simulink model "drone_HyEQ"  (R2025b)
settings: Solver=VariableStepAuto  StartTime=0.0  StopTime=T  RelTol=1e-3
values from neighbouring files (symbols this model uses):
  J = 100    [init.m]
  T = 100    [init.m]
  x0 = zeros(14,1)    [init.m]
libraries: HyEQ_Library x2, simulink_extras x1
settings Model: Creator=jenniferkouassi  LastModifiedBy=jenniferkouassi
settings DebuggingCC: AlgebraicLoopMsg=none

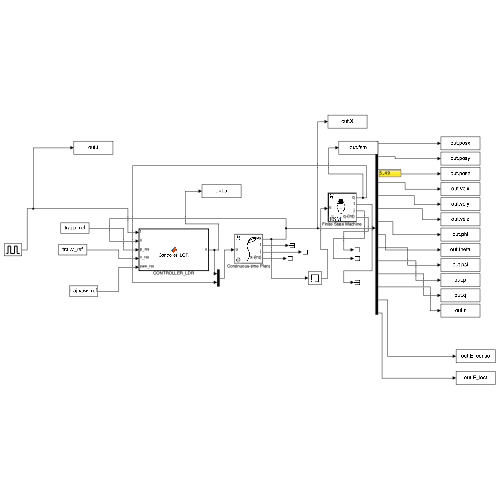
[thumbnail: Simulink's stored preview of the top-level diagram]
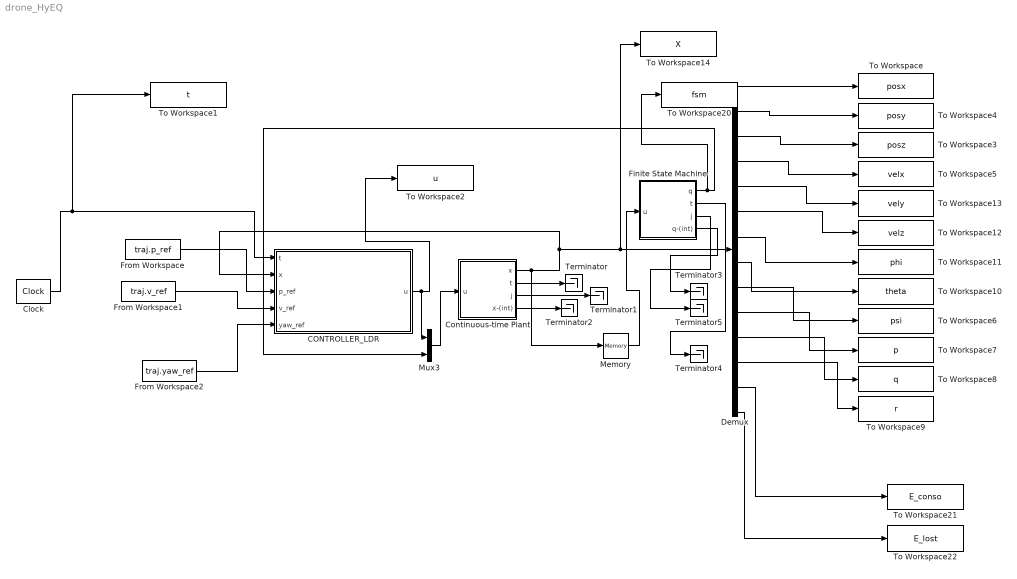
== system drone_HyEQ ==
  CONTROLLER_LDR : MATLAB Function  TreatAsAtomicUnit=on
  Clock : simulink_extras/Flip Flops/Clock  period=120
  Continuous-time Plant : Subsystem  LoadFcn=set_param(gcb,'LinkStatus','none')  mask(Continuous Process){z0=x0, input_dim=[5, 1], parameters=[], T=T}
      mask prompts: z0 "Initial State (column vector)"; input_dim "Input dimension (nonnegative integer)"; T "Flow Horizon (nonnegative real)"
      mask help:
      | To define the continuous process:
      | 1. Select the block,
      | 2. "Look inside" the block: Either open the context menu and select Mask > Look Under Mask, or click the arrow in the bottom-left corner of the block.
      | 3. Edit the "flow map f" block to define the continuous dynamics.
      | 4. Edit the "flow set C" block to define the region where the continuous process is allowed to flow.
      mask init:
      | state_dim = size(z0, 1);
      settings: CopyFcn=|
      | set_param(gcb,'LinkStatus','none'),
      | set_param(gcs, 'MaxStep', 'MaxStep', 'RelTol', 'RelTol','StopTime', 'T')
      mask Help: eval hybrid.internal.openHelp('Example_vehicle_on_path')
      mask TypeOptions T: Integrator System/T
      mask DialogControl Control2 Prompt: CPS Components Documentation
      mask DialogControl Control2 Callback: hybrid.internal.openHelp('CPS_Components')
      mask DialogControl ParameterGroupVar Prompt: Configuration
      mask Display:
      | image('Cplant.jpg')
      | port_label('output', 1, 'x')
      | port_label('output', 2, 't')
      | port_label('output', 3, 'j')
      | port_label('output', 4, 'x-(int)')
      | port_label('input', 1, 'u')
  Demux : Demux  Outputs=14
  Finite State Machine : Subsystem  LoadFcn=set_param(gcb,'LinkStatus','none')  mask(Finite State Machine (FSM)){q0=1, input_dim=14, T=T, J=J}
      mask prompts: q0 "Initial state (column vector)"; input_dim "Input dimension (nonnegative integer)"; T "Flow Horizon (nonnegative real)"; J "Jump Horizon (nonnegative integer)"
      mask help:
      | To define the FSM:
      | 1. Select the block,
      | 2. "Look inside" the block: Either open the context menu and select Mask > Look Under Mask, or click the arrow in the bottom-left corner of the block.
      | 3. Edit the flow set C, jump set D, and jump map g.
      mask init:
      | state_dim = numel(q0);
      settings: CopyFcn=|
      | set_param(gcb,'LinkStatus','none'),
      | set_param(gcs, 'MaxStep', 'MaxStep', 'RelTol', 'RelTol','StopTime', 'T')
      mask Help: eval hybrid.internal.openHelp('CPS_finite_state_machine')
      mask TypeOptions T: Integrator System/T
      mask TypeOptions J: Integrator System/J
      mask DialogControl Control2 Prompt: CPS Components Documentation
      mask DialogControl Control2 Callback: hybrid.internal.openHelp('CPS_Components')
      mask DialogControl Container4 Prompt: Configuration
      mask Display:
      | image('FSM.jpg')
      | port_label('output', 1, 'q')
      | port_label('output', 2, 't')
      | port_label('output', 3, 'j')
      | port_label('output', 4, 'q-(int)')
      | port_label('input', 1, 'u')
  From Workspace : FromWorkspace  VariableName=traj.p_ref  OutputAfterFinalValue=Holding final value
  From Workspace1 : FromWorkspace  VariableName=traj.v_ref  OutputAfterFinalValue=Holding final value
  From Workspace2 : FromWorkspace  VariableName=traj.yaw_ref
  Memory : Memory
  Mux3 : Mux  Inputs=2
  Terminator{,1..5} (6 alike) : Terminator
  To Workspace : ToWorkspace  VariableName=posx  SaveFormat=Timeseries
  To Workspace1 : ToWorkspace  VariableName=t  SaveFormat=Timeseries
  To Workspace10 : ToWorkspace  VariableName=theta  SaveFormat=Timeseries
  To Workspace11 : ToWorkspace  VariableName=phi  SaveFormat=Timeseries
  To Workspace12 : ToWorkspace  VariableName=velz  SaveFormat=Timeseries
  To Workspace13 : ToWorkspace  VariableName=vely  SaveFormat=Timeseries
  To Workspace14 : ToWorkspace  VariableName=X  SaveFormat=Timeseries
  To Workspace2 : ToWorkspace  VariableName=u  SaveFormat=Timeseries
      settings: Save2DSignal=2-D array (concatenate along first dimension)
  To Workspace20 : ToWorkspace  VariableName=fsm  SaveFormat=Timeseries  SampleTime=-1
      settings: Save2DSignal=2-D array (concatenate along first dimension)
  To Workspace21 : ToWorkspace  VariableName=E_conso  SaveFormat=Timeseries  SampleTime=-1
      settings: Save2DSignal=2-D array (concatenate along first dimension)
  To Workspace22 : ToWorkspace  VariableName=E_lost  SaveFormat=Timeseries  SampleTime=-1
      settings: Save2DSignal=2-D array (concatenate along first dimension)
  To Workspace3 : ToWorkspace  VariableName=posz  SaveFormat=Timeseries
  To Workspace4 : ToWorkspace  VariableName=posy  SaveFormat=Timeseries
      settings: Save2DSignal=2-D array (concatenate along first dimension)
  To Workspace5 : ToWorkspace  VariableName=velx  SaveFormat=Timeseries
  To Workspace6 : ToWorkspace  VariableName=psi  SaveFormat=Timeseries
  To Workspace7 : ToWorkspace  VariableName=p  SaveFormat=Timeseries
  To Workspace8 : ToWorkspace  VariableName=q  SaveFormat=Timeseries
  To Workspace9 : ToWorkspace  VariableName=r  SaveFormat=Timeseries
  wires:
  Clock/1 -> To Workspace1/1, CONTROLLER_LDR/1(t)
  Continuous-time Plant/1(x) -> Memory/1, CONTROLLER_LDR/2(x), To Workspace14/1, Demux/1
  From Workspace/1 -> CONTROLLER_LDR/3(p_ref)
  From Workspace1/1 -> CONTROLLER_LDR/4(v_ref)
  From Workspace2/1 -> CONTROLLER_LDR/5(yaw_ref)
  CONTROLLER_LDR/1(u) -> Mux3/1, To Workspace2/1
  Continuous-time Plant/2(t) -> Terminator/1
  Continuous-time Plant/3(j) -> Terminator1/1
  Continuous-time Plant/4(x-(int)) -> Terminator2/1
  Demux/12 -> To Workspace9/1
  Demux/11 -> To Workspace8/1
  Demux/10 -> To Workspace7/1
  Demux/9 -> To Workspace6/1
  Demux/8 -> To Workspace10/1
  Demux/7 -> To Workspace11/1
  Demux/6 -> To Workspace12/1
  Demux/5 -> To Workspace13/1
  Demux/4 -> To Workspace5/1
  Demux/3 -> To Workspace3/1
  Demux/2 -> To Workspace4/1
  Demux/1 -> To Workspace/1
  Finite State Machine/4(q-(int)) -> Terminator3/1
  Finite State Machine/3(j) -> Terminator5/1
  Finite State Machine/2(t) -> Terminator4/1
  Finite State Machine/1(q) -> To Workspace20/1, Mux3/2
  Mux3/1 -> Continuous-time Plant/1(u)
  Memory/1 -> Finite State Machine/1(u)
  Demux/13 -> To Workspace21/1
  Demux/14 -> To Workspace22/1

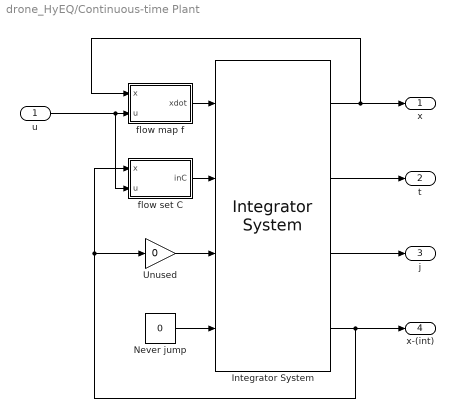
== system drone_HyEQ/Continuous-time Plant ==
  u : Inport  PortDimensions=input_dim
  Integrator System : HyEQ_Library/Other/Integrator System  Priority=2  T=T  J=1  x0=z0  rule=1
      settings: SourceProductName=Hybrid Equations Toolbox
  Never jump : Constant  Value=0
  Unused : Gain  Gain=0
  flow map f : MATLAB Function  TreatAsAtomicUnit=on
  flow set C : MATLAB Function  TreatAsAtomicUnit=on
  x : Outport  PortDimensions=state_dim
  t : Outport  Port=2  PortDimensions=1
  j : Outport  Port=3  PortDimensions=1
  x-(int) : Outport  Port=4  PortDimensions=state_dim
  wires:
  Unused/1 -> Integrator System/3
  Never jump/1 -> Integrator System/4
  u/1 -> flow map f/2(u), flow set C/2(u)
  Integrator System/3 -> j/1
  Integrator System/2 -> t/1
  flow set C/1(inC) -> Integrator System/2
  Integrator System/1 -> x/1, flow map f/1(x)
  Integrator System/4 -> x-(int)/1, flow set C/1(x), Unused/1
  flow map f/1(xdot) -> Integrator System/1

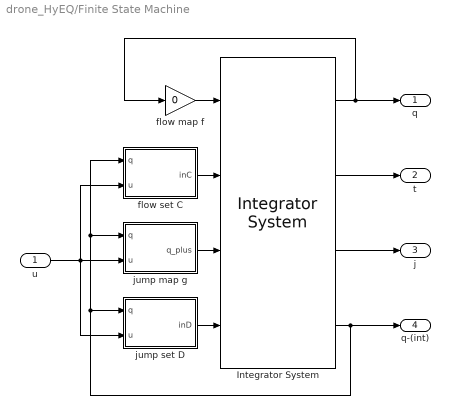
== system drone_HyEQ/Finite State Machine ==
  u : Inport  PortDimensions=input_dim
  Integrator System : HyEQ_Library/Other/Integrator System  Priority=2  T=T  J=J  x0=q0  rule=1
      settings: SourceProductName=Hybrid Equations Toolbox
  flow map f : Gain  Gain=0
  flow set C : MATLAB Function  TreatAsAtomicUnit=on
  jump map g : MATLAB Function  TreatAsAtomicUnit=on
  jump set D : MATLAB Function  TreatAsAtomicUnit=on
  q : Outport  PortDimensions=state_dim
  t : Outport  Port=2  PortDimensions=1
  j : Outport  Port=3  PortDimensions=1
  q-(int) : Outport  Port=4  PortDimensions=state_dim
  wires:
  jump map g/1(q_plus) -> Integrator System/3
  jump set D/1(inD) -> Integrator System/4
  u/1 -> jump map g/2(u), jump set D/2(u), flow set C/2(u)
  Integrator System/3 -> j/1
  Integrator System/2 -> t/1
  flow set C/1(inC) -> Integrator System/2
  Integrator System/1 -> q/1, flow map f/1
  Integrator System/4 -> q-(int)/1, flow set C/1(q), jump map g/1(q), jump set D/1(q)
  flow map f/1 -> Integrator System/1

== matlab function drone_HyEQ/CONTROLLER_LDR ==
  data: t input; u output size=[4, 1]; x input; p_ref input; v_ref input; yaw_ref input; P parameter
function u = Controller_LQR(t, x, p_ref, v_ref, yaw_ref, P)
%CONTROLLER_LQR Cascaded LQR controller for quadcopter
%   x   = [px py pz vx vy vz phi theta psi p q r]'
%   P   = parameter struct (contains precomputed K_pos and K_att)

%% --- Outer loop: Position control (x,y) -> desired accelerations ---
x_pos = x(1:6);
xr_pos = [p_ref; v_ref];

% Calcul de l'accélération désirée pour x et y avec LQR
u_pos = -P.K_pos * (x_pos - xr_pos);

%% --- Contrôle vertical (évite la chute) ---
z    = x(3);      % position actuelle
vz   = x(6);      % vitesse verticale
zref = p_ref(3);  % position désirée
vzref = v_ref(3); % vitesse désirée

Kpz = 6;          % gain proportionnel vertical
Kdz = 3;          % gain dérivé vertical
az_des = Kpz*(zref - z) + Kdz*(vzref - vz);  % accélération verticale désirée

F_total = P.m * (P.g + az_des);              % poussée totale (hover + correction)
F_total = min(max(F_total, 0), 3*P.m*P.g);   % limite pour éviter la saturation

%% --- Map desired acceleration to desired roll/pitch ---
psi = x(9);
phi_des   = (1/P.g) * (u_pos(1)*sin(psi) - u_pos(2)*cos(psi));
theta_des = (1/P.g) * (u_pos(1)*cos(psi) + u_pos(2)*sin(psi));

%% --- Inner loop: Attitude control (phi, theta, psi) -> torques ---
x_att = x(7:12);
xr_att = [phi_des; theta_des; yaw_ref; 0; 0; 0];
tau = -P.K_att * (x_att - xr_att);

% Saturation des couples
tau = max(min(tau, P.tau_max), -P.tau_max);

%% --- Sortie du contrôleur ---
u = [F_total; tau];

end

== matlab function drone_HyEQ/Finite State Machine/flow set C ==
  data: q input size=state_dim; u input size=input_dim; inC output size=1
function inC = C(q, u)

% Force q to be an exact integer but KEEP IT DOUBLE
q = round(q);

alt = u(3);

switch q
    case 1
        inC = (alt <= 1.5);

    case 2
        inC = (alt > 0.5 && alt <= 2.5);

    case 3
        inC = (alt > 1.5 && alt <= 4.0);

    case 4
        inC = (alt > 2.5);

    otherwise
        inC = false;
end

end

== matlab function drone_HyEQ/Finite State Machine/jump map g ==
  data: q input size=state_dim; u input size=input_dim; q_plus output size=state_dim
function q_plus = g(q, u)

% Ensure q is integer-valued but REMAINING double
q = round(q);

alt = u(3);

switch q

    case 1
        q_plus = 2;

    case 2
        if alt > 1.5
            q_plus = 3;
        else
            q_plus = 1;
        end

    case 3
        if alt > 3.0
            q_plus = 4;
        else
            q_plus = 2;
        end

    case 4
        if alt < 2.5
            q_plus = 3;
        else
            q_plus = 4;
        end

    otherwise
        q_plus = 1;

end

end

== matlab function drone_HyEQ/Finite State Machine/jump set D ==
  data: q input size=state_dim; u input size=input_dim; inD output size=1
function inD = D(q, u)

% Keep q DOUBLE but integer-valued
q = round(q);

alt = u(3);

switch q
    case 1
        inD = (alt > 1.0);

    case 2
        inD = (alt > 2.0);

    case 3
        inD = (alt > 3.0);

    case 4
        inD = (alt < 2.0);

    otherwise
        inD = false;
end

end

== matlab function drone_HyEQ/Continuous-time Plant/flow map f ==
  data: x input size=state_dim; xdot output size=state_dim; u input size=input_dim; P parameter
function xdot = f(x, u, P)
% DYNAMIQUE COMPLETE DU DRONE
% AVEC TRAÎNÉE MULTI-SURFACES + COUPLES AÉRODYNAMIQUES + ÉNERGIE

%% === 1. Décomposition des entrées ===
u_cmd = u(1:4);    % [u1 ; tau_x ; tau_y ; tau_z]
mode_FSM = u(5);   % q = 1 → calme, 2 → vent léger, 3 → rafales, 4 → tempête

%% === 2. Vent selon FSM (déterministe, pas de randn) ===
%% === 2. Vent selon FSM (4 niveaux : calme → tempête) ===

pos_x = x(1);
pos_y = x(2);
pos_z = x(3);

% Turbulence pseudo-aléatoire déterministe (pas de randn)
rafale_x =  1.2 * sin(0.6 * pos_x) + 0.8 * cos(1.1 * pos_y);
rafale_y =  0.6 * sin(0.9 * pos_y) + 0.5 * cos(1.3 * pos_z);
rafale_z =  0.3 * sin(0.5 * pos_z) + 0.3 * cos(0.7 * pos_x);

switch mode_FSM      % q = 1 / 2 / 3 / 4

    case 1  % --- Calme ---
        V_air = [0; 0; 0];

    case 2  % --- Vent léger ---
        V_air = [ 3 + 0.4*rafale_x ;
                  0.5*rafale_y ;
                  0.2*rafale_z ];

    case 3  % --- Rafales modérées ---
        V_air = [ 6 + 1.2*rafale_x ;
                      1*rafale_y ;
                  0.6*rafale_z ];

    case 4  % --- Tempête ---
        V_air = [ 10 + 2.0*rafale_x ;
                        2*rafale_y ;
                        1*rafale_z ];

    otherwise
        V_air = [0;0;0];

end

%% === 3. États ===
vx = x(4); vy = x(5); vz = x(6);
phi = x(7); theta = x(8); psi = x(9);
p = x(10); q = x(11); r = x(12);

V_drone = [vx; vy; vz];
V_rel   = V_air - V_drone;     % vitesse du vent relative

%% === 4. Aérodynamique multisurface (forces + moments) ===
F_vent = [0; 0; 0];
M_vent = [0; 0; 0];

%% --- Face avant (X+) ---
Vn = V_rel(1);
F = -0.5 * P.rho * P.Sx_front * P.Cd * Vn * abs(Vn) * [1;0;0];
F_vent = F_vent + F;
M_vent = M_vent + cross(P.r_cp_x, F);

%% --- Face arrière (X−) ---
Vn = -V_rel(1);
F = -0.5 * P.rho * P.Sx_back * P.Cd * Vn * abs(Vn) * [-1;0;0];
F_vent = F_vent + F;
M_vent = M_vent + cross(P.r_cp_mx, F);

%% --- Face droite (Y+) ---
Vn = V_rel(2);
F = -0.5 * P.rho * P.Sy_right * P.Cd * Vn * abs(Vn) * [0;1;0];
F_vent = F_vent + F;
M_vent = M_vent + cross(P.r_cp_y, F);

%% --- Face gauche (Y−) ---
Vn = -V_rel(2);
F = -0.5 * P.rho * P.Sy_left * P.Cd * Vn * abs(Vn) * [0;-1;0];
F_vent = F_vent + F;
M_vent = M_vent + cross(P.r_cp_my, F);

%% --- Face dessus (Z+) ---
Vn = V_rel(3);
F = -0.5 * P.rho * P.Sz_top * P.Cd * Vn * abs(Vn) * [0;0;1];
F_vent = F_vent + F;
M_vent = M_vent + cross(P.r_cp_z, F);

%% --- Face dessous (Z−) ---
Vn = -V_rel(3);
F = -0.5 * P.rho * P.Sz_bottom * P.Cd * Vn * abs(Vn) * [0;0;-1];
F_vent = F_vent + F;
M_vent = M_vent + cross(P.r_cp_mz, F);

%% === 5. Rotation (matrice R du corps vers monde) ===
cphi = cos(phi);  sphi = sin(phi);
cth  = cos(theta); sth  = sin(theta);
cpsi = cos(psi);  spsi = sin(psi);

R = [ cth*cpsi,  sphi*sth*cpsi - cphi*spsi,  cphi*sth*cpsi + sphi*spsi;
      cth*spsi,  sphi*sth*spsi + cphi*cpsi,  cphi*sth*spsi - sphi*cpsi;
     -sth,       sphi*cth,                  cphi*cth ];

%% === 6. Translation ===
u1 = u_cmd(1);

p_dot = [vx; vy; vz];

v_dot = (1/P.m) * (R*[0;0;u1] + F_vent) - [0;0;P.g];

%% === 7. Angles ===
E = [1,  sphi*tan(theta),  cphi*tan(theta);
     0,  cphi,            -sphi;
     0,  sphi/cth,         cphi/cth];

eul_dot = E * [p; q; r];

%% === 8. Rotation + couples du vent ===
I = P.I;
omega = [p; q; r];
tau = u_cmd(2:4);

omega_dot = I \ (tau + M_vent - cross(omega, I*omega));

%% === 9. Énergie ===
u1_safe = max(u1, 0);
Omega = sqrt(u1_safe / (4*P.kf));
Couple_tot = 4 * P.km * Omega^2;

P_meca = Couple_tot * Omega;
P_elec_dot = (P_meca / P.eta) + P.E_sub;

P_lost_dot = abs(dot(F_vent, V_drone));

%% === 10. Output final ===
xdot = [
    p_dot;
    v_dot;
    eul_dot;
    omega_dot;
    P_elec_dot;
    P_lost_dot
];

end

== matlab function drone_HyEQ/Continuous-time Plant/flow set C ==
  data: x input size=state_dim; inC output size=1; u input size=input_dim
function inC = C(x, u)
    % Define the flow set indicator function for the continuous process here.
    inC = 1;
end
